simulink model "FSAE"  (R2023a)
settings: Solver=VariableStepAuto  StartTime=0.0  StopTime=1220  RelTol=1e-3
undefined symbols (not defined in the file): eta_EM_map, g, h, r_wheel, rho, T_EM_max, w_EM_row, w_EM_upper
settings Model: Creator=123ne  LastModifiedBy=123ne
settings ModelReferenceCC: EnableRefExpFcnMdlSchedulingChecks=on

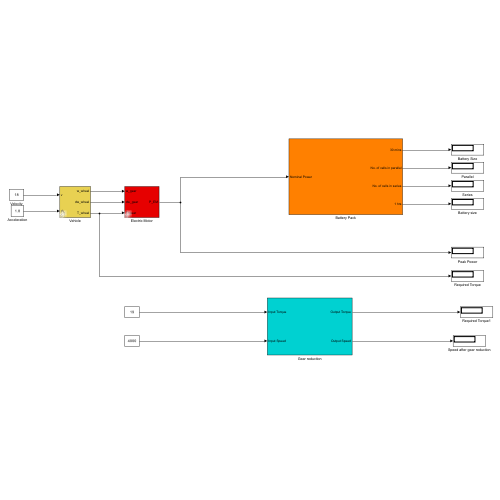
[thumbnail: Simulink's stored preview of the top-level diagram]
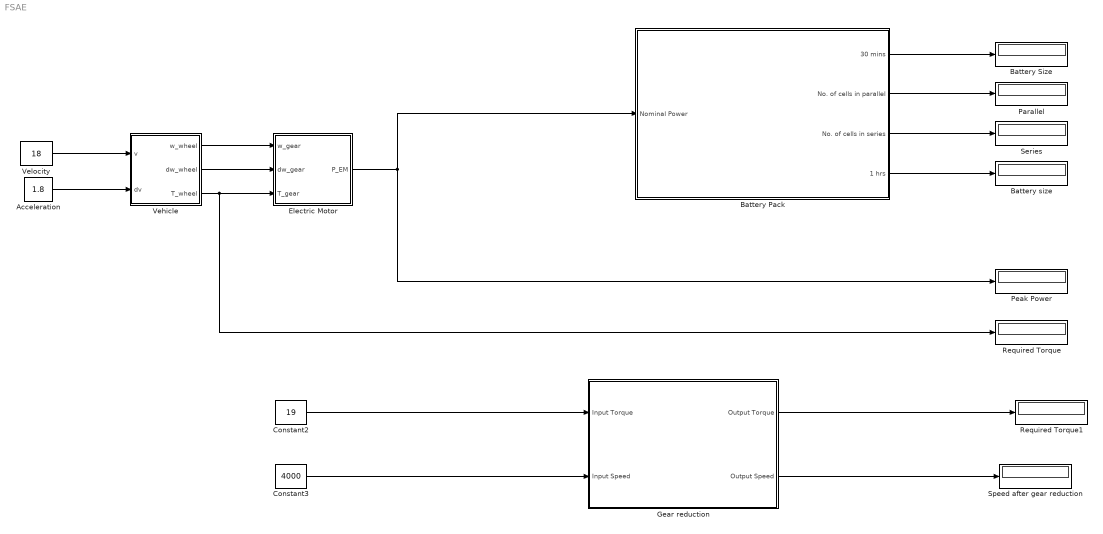
== system FSAE ==
  Acceleration : Constant  Value=1.8
  Battery Pack : Subsystem  mask{V_u=72, V_n=3.7}
      mask prompts: V_u "Specified Voltage"; V_n "Nominal Voltage"
  Battery Size : Display
  Battery size : Display
  Constant2 : Constant  Value=19
  Constant3 : Constant  Value=4000
  Electric Motor : Subsystem  AncestorBlock=qss_tb_library/Energy Converter/Electric Motor  mask(Electric Motor){scale_EM=1, theta_EM=0.1, P_aux=0}
      mask prompts: scale_EM "Motor scaling factor [-]"; theta_EM "Motor inertia [kg*m2]"; P_aux "Power required by auxiliaries [W]"
      mask help:
      | This block simulates the behaviour of an electric motor. The block is based on an efficiency map.
      |
      | Input:
      | =====
      | 	w_gear		Speed of the fly wheel [rad/s]
      | 	dw_gear	Acceleration of the fly wheel [rad/s^2]
      | 	T_gear		Torque on the fly wheel [Nm]
      |
      | Output:
      | ======
      | 	P_EM		Power produced by the electric motor [W]
      mask init:
      | init_EM;
      settings: LibrarySourceBlock=qss_tb_library/Energy Converter/Electric Motor
  Gear reduction : Subsystem  mask{r1=3.14, r2=4, r_1=3.14, r_2=4, R=0.507}
      mask prompts: r1 "Gear ratio"; r2 "Differential ratio"; r_1 "Gear ratio1"; r_2 "Differential ratio2"; R "radius"
  Parallel : Display
  Peak Power : Display
  Required Torque : Display
  Required Torque1 : Display
  Series : Display
  Speed after gear reduction : Display
  Vehicle : Subsystem  Tag=vehicle  AncestorBlock=qss_tb_library/Vehicle/Vehicle  mask(Vehicle){m_f=350, mt2m_f=5, A_f=0.35, d_wheel=0.507, cw=0.85, mu=0.018}
      mask prompts: m_f "Total mass of the vehicle [kg]"; mt2m_f "Rotating mass [%]"; A_f "Vehicle cross section [m^2]"; d_wheel "Wheel diameter [m]"; cw "Drag coefficient [-]"; mu "Rolling friction coefficient [-]"
      mask help:
      | This block computes the power required from the vehicle.
      |
      | Input:
      | =====
      | 	v		Speed [m/s]
      | 	dv		Acceleration [m/s^2]
      |
      | Output:
      | ======
      | 	w_wheel	Speed of the wheel [rad/s]
      | 	dw_wheel	Acceleration of the wheel [rad/s^2]
      | 	T_wheel	Torque on the wheel [Nm]
      mask init:
      | init_vehicle;
      settings: LibrarySourceBlock=qss_tb_library/Vehicle/Vehicle
  Velocity : Constant  Value=18
  wires:
  Vehicle/1(w_wheel) -> Electric Motor/1(w_gear)
  Vehicle/2(dw_wheel) -> Electric Motor/2(dw_gear)
  Vehicle/3(T_wheel) -> Electric Motor/3(T_gear), Required Torque/1
  Battery Pack/1(30 mins) -> Battery Size/1
  Battery Pack/2(No. of cells in parallel) -> Parallel/1
  Battery Pack/3(No. of cells in series) -> Series/1
  Battery Pack/4(1 hrs) -> Battery size/1
  Electric Motor/1(P_EM) -> Battery Pack/1(Nominal Power), Peak Power/1
  Constant2/1 -> Gear reduction/1(Input Torque)
  Gear reduction/1(Output Torque) -> Required Torque1/1
  Constant3/1 -> Gear reduction/2(Input Speed)
  Gear reduction/2(Output Speed) -> Speed after gear reduction/1
  Velocity/1 -> Vehicle/1(v)
  Acceleration/1 -> Vehicle/2(dv)

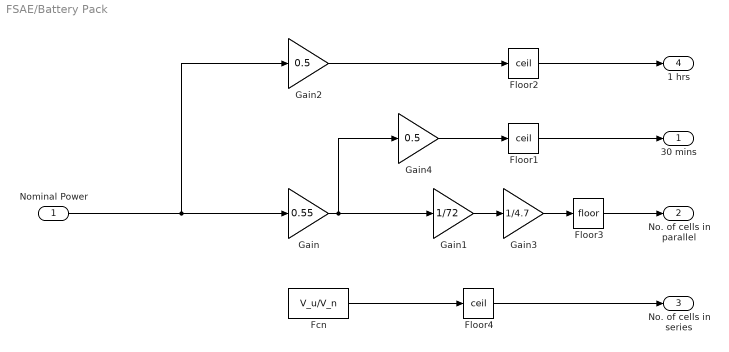
== system FSAE/Battery Pack ==
  Nominal Power : Inport
  Fcn : Fcn  Expr=V_u/V_n
  Floor1 : Rounding  Operator=ceil
  Floor2 : Rounding  Operator=ceil
  Floor3 : Rounding
  Floor4 : Rounding  Operator=ceil
  Gain : Gain  Gain=0.55
  Gain1 : Gain  Gain=1/72
  Gain2 : Gain  Gain=0.5
  Gain3 : Gain  Gain=1/4.7
  Gain4 : Gain  Gain=0.5
  30 mins : Outport
  No. of cells in parallel : Outport  Port=2
  No. of cells in series : Outport  Port=3
  1 hrs : Outport  Port=4
  wires:
  Gain/1 -> Gain1/1, Gain4/1
  Nominal Power/1 -> Gain2/1, Gain/1
  Gain1/1 -> Gain3/1
  Gain3/1 -> Floor3/1
  Floor1/1 -> 30 mins/1
  Fcn/1 -> Floor4/1
  Floor3/1 -> No. of cells in parallel/1
  Floor4/1 -> No. of cells in series/1
  Gain2/1 -> Floor2/1
  Floor2/1 -> 1 hrs/1
  Gain4/1 -> Floor1/1

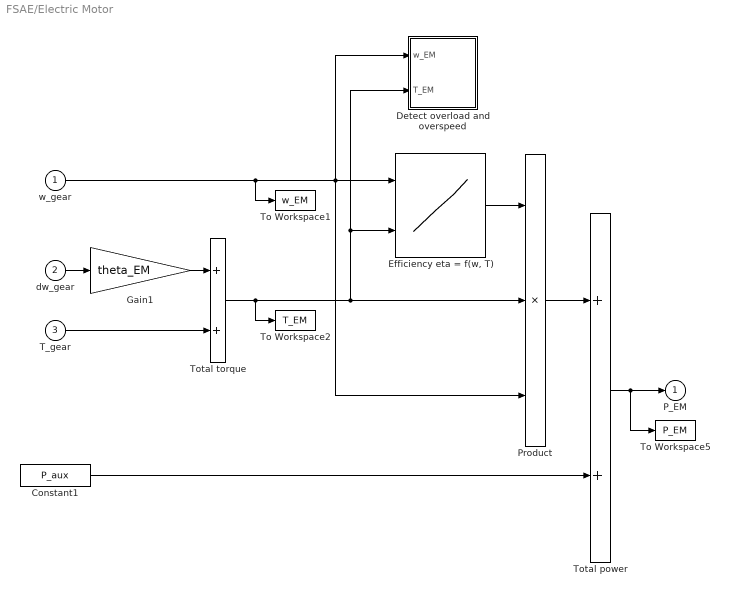
== system FSAE/Electric Motor ==
  w_gear : Inport
  dw_gear : Inport  Port=2
  T_gear : Inport  Port=3
  Constant1 : Constant  Value=P_aux
  Detect overload and overspeed : Subsystem
  "Efficiency eta = f(w, T)" : Lookup2D  RowIndex=w_EM_row  ColumnIndex=T_EM_col  Table=eta_EM_map  SaturateOnIntegerOverflow=off  InputSameDT=off
  Gain1 : Gain  Gain=theta_EM  SaturateOnIntegerOverflow=on  OutDataTypeStr=Inherit: Same as input  ParamDataTypeStr=Inherit: Same as input
  Product : Product  Inputs=3  InputSameDT=on  RndMeth=Zero  SaturateOnIntegerOverflow=on  OutDataTypeStr=Inherit: Same as first input
  To Workspace1 : ToWorkspace  VariableName=w_EM  SampleTime=-1
  To Workspace2 : ToWorkspace  VariableName=T_EM  SampleTime=-1
  To Workspace5 : ToWorkspace  VariableName=P_EM  SampleTime=-1
  Total power : Sum  InputSameDT=on  SaturateOnIntegerOverflow=on  OutDataTypeStr=Inherit: Same as first input
  Total torque : Sum  InputSameDT=on  SaturateOnIntegerOverflow=on  OutDataTypeStr=Inherit: Same as first input
  P_EM : Outport  InitialOutput=0
  wires:
  Total power/1 -> To Workspace5/1, P_EM/1
  Product/1 -> Total power/1
  Constant1/1 -> Total power/2
  Total torque/1 -> Product/2, "Efficiency eta = f(w, T)"/2, Detect overload and overspeed/2(T_EM), To Workspace2/1
  Gain1/1 -> Total torque/1
  T_gear/1 -> Total torque/2
  dw_gear/1 -> Gain1/1
  "Efficiency eta = f(w, T)"/1 -> Product/1
  w_gear/1 -> To Workspace1/1, Product/3, "Efficiency eta = f(w, T)"/1, Detect overload and overspeed/1(w_EM)

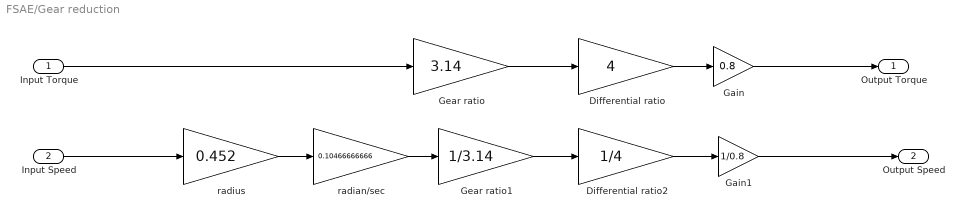
== system FSAE/Gear reduction ==
  Input Torque : Inport
  Input Speed : Inport  Port=2
  Differential ratio : Gain  Gain=4
  Differential ratio2 : Gain  Gain=1/4
  Gain : Gain  Gain=0.8
  Gain1 : Gain  Gain=1/0.8
  Gear ratio : Gain  Gain=3.14
  Gear ratio1 : Gain  Gain=1/3.14
  radian/sec : Gain  Gain=0.10466666666
  radius : Gain  Gain=0.452
  Output Torque : Outport
  Output Speed : Outport  Port=2
  wires:
  Gear ratio1/1 -> Differential ratio2/1
  Gear ratio/1 -> Differential ratio/1
  Input Torque/1 -> Gear ratio/1
  Input Speed/1 -> radius/1
  Differential ratio/1 -> Gain/1
  Differential ratio2/1 -> Gain1/1
  radius/1 -> radian/sec/1
  radian/sec/1 -> Gear ratio1/1
  Gain/1 -> Output Torque/1
  Gain1/1 -> Output Speed/1

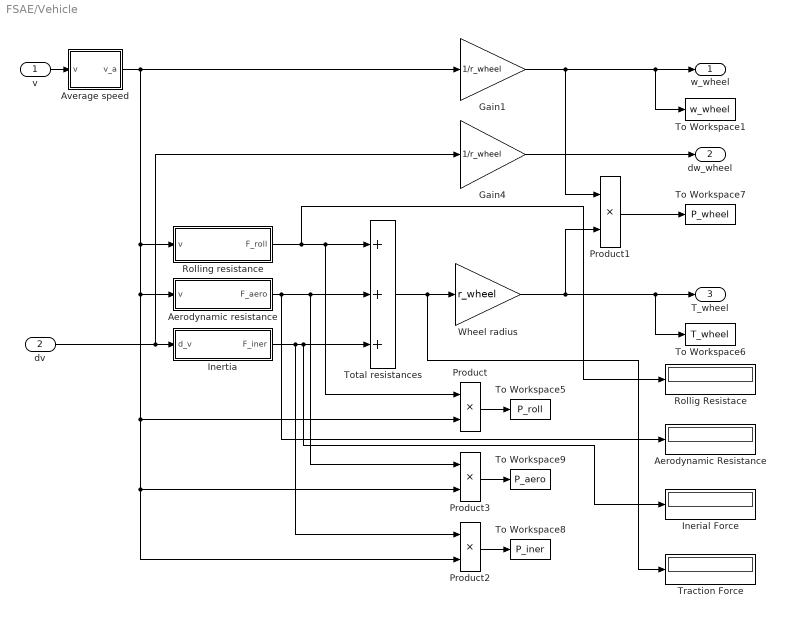
== system FSAE/Vehicle ==
  v : Inport
  dv : Inport  Port=2
  Aerodynamic Resistance : Display
  Aerodynamic resistance : Subsystem
  Average speed : Subsystem
  Gain1 : Gain  Gain=1/r_wheel  SaturateOnIntegerOverflow=on  OutDataTypeStr=Inherit: Same as input  ParamDataTypeStr=Inherit: Same as input
  Gain4 : Gain  Gain=1/r_wheel  SaturateOnIntegerOverflow=on  OutDataTypeStr=Inherit: Same as input  ParamDataTypeStr=Inherit: Same as input
  Inerial Force : Display
  Inertia : Subsystem
  Product{,1..3} (4 alike) : Product  InputSameDT=on  RndMeth=Zero  SaturateOnIntegerOverflow=on  OutDataTypeStr=Inherit: Same as first input
  Rollig Resistace : Display
  Rolling resistance : Subsystem
  To Workspace1 : ToWorkspace  VariableName=w_wheel  SampleTime=-1
  To Workspace5 : ToWorkspace  VariableName=P_roll  SampleTime=-1
  To Workspace6 : ToWorkspace  VariableName=T_wheel  SampleTime=-1
  To Workspace7 : ToWorkspace  VariableName=P_wheel  SampleTime=-1
  To Workspace8 : ToWorkspace  VariableName=P_iner  SampleTime=-1
  To Workspace9 : ToWorkspace  VariableName=P_aero  SampleTime=-1
  Total resistances : Sum  Inputs=+++  InputSameDT=on  SaturateOnIntegerOverflow=on  OutDataTypeStr=Inherit: Same as first input
  Traction Force : Display
  Wheel radius : Gain  Gain=r_wheel  SaturateOnIntegerOverflow=on  OutDataTypeStr=Inherit: Same as input  ParamDataTypeStr=Inherit: Same as input
  w_wheel : Outport  InitialOutput=0
  dw_wheel : Outport  Port=2  InitialOutput=0
  T_wheel : Outport  Port=3  InitialOutput=0
  wires:
  Product/1 -> To Workspace5/1
  Product1/1 -> To Workspace7/1
  Product3/1 -> To Workspace9/1
  Product2/1 -> To Workspace8/1
  v/1 -> Average speed/1(v)
  dv/1 -> Gain4/1, Inertia/1(d_v)
  Average speed/1(v_a) -> Rolling resistance/1(v), Product2/2, Product3/2, Product/2, Aerodynamic resistance/1(v), Gain1/1
  Wheel radius/1 -> To Workspace6/1, T_wheel/1, Product1/2
  Total resistances/1 -> Traction Force/1, Wheel radius/1
  Inertia/1(F_iner) -> Product2/1, Inerial Force/1, Total resistances/3
  Aerodynamic resistance/1(F_aero) -> Aerodynamic Resistance/1, Total resistances/2, Product3/1
  Rolling resistance/1(F_roll) -> Rollig Resistace/1, Product/1, Total resistances/1
  Gain1/1 -> To Workspace1/1, w_wheel/1, Product1/1
  Gain4/1 -> dw_wheel/1

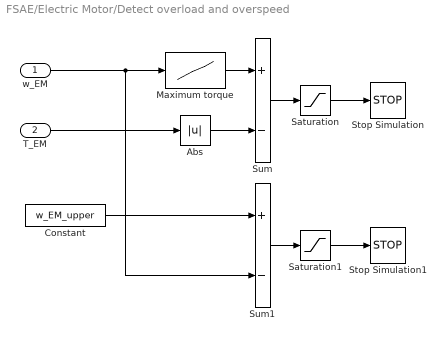
== system FSAE/Electric Motor/Detect overload and overspeed ==
  w_EM : Inport
  T_EM : Inport  Port=2
  Abs : Abs
  Constant : Constant  Value=w_EM_upper
  Maximum torque : Lookup  InputValues=w_EM_row  Table=T_EM_max
  Saturation : Saturate  UpperLimit=0  LowerLimit=-inf
  Saturation1 : Saturate  UpperLimit=0  LowerLimit=-inf
  Stop Simulation : Stop
  Stop Simulation1 : Stop
  Sum : Sum  Inputs=+-  InputSameDT=on  SaturateOnIntegerOverflow=on  OutDataTypeStr=Inherit: Same as first input
  Sum1 : Sum  Inputs=+-  InputSameDT=on  SaturateOnIntegerOverflow=on  OutDataTypeStr=Inherit: Same as first input
  wires:
  Sum/1 -> Saturation/1
  w_EM/1 -> Maximum torque/1, Sum1/2
  T_EM/1 -> Abs/1
  Maximum torque/1 -> Sum/1
  Abs/1 -> Sum/2
  Saturation/1 -> Stop Simulation/1
  Constant/1 -> Sum1/1
  Sum1/1 -> Saturation1/1
  Saturation1/1 -> Stop Simulation1/1

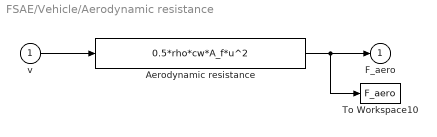
== system FSAE/Vehicle/Aerodynamic resistance ==
  v : Inport
  Aerodynamic resistance : Fcn  Expr=0.5*rho*cw*A_f*u^2
  To Workspace10 : ToWorkspace  VariableName=F_aero  SampleTime=-1
  F_aero : Outport  InitialOutput=0
  wires:
  Aerodynamic resistance/1 -> To Workspace10/1, F_aero/1
  v/1 -> Aerodynamic resistance/1

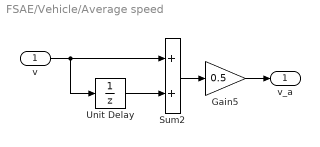
== system FSAE/Vehicle/Average speed ==
  v : Inport
  Gain5 : Gain  Gain=0.5  SaturateOnIntegerOverflow=on  OutDataTypeStr=Inherit: Same as input  ParamDataTypeStr=Inherit: Same as input
  Sum2 : Sum  InputSameDT=on  SaturateOnIntegerOverflow=on  OutDataTypeStr=Inherit: Same as first input
  Unit Delay : UnitDelay  SampleTime=h
  v_a : Outport  InitialOutput=0
  wires:
  v/1 -> Unit Delay/1, Sum2/1
  Gain5/1 -> v_a/1
  Sum2/1 -> Gain5/1
  Unit Delay/1 -> Sum2/2

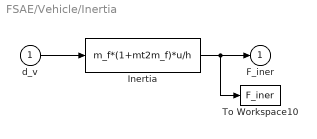
== system FSAE/Vehicle/Inertia ==
  d_v : Inport
  Inertia : Fcn  Expr=m_f*(1+mt2m_f)*u/h
  To Workspace10 : ToWorkspace  VariableName=F_iner  SampleTime=-1
  F_iner : Outport  InitialOutput=0
  wires:
  d_v/1 -> Inertia/1
  Inertia/1 -> To Workspace10/1, F_iner/1

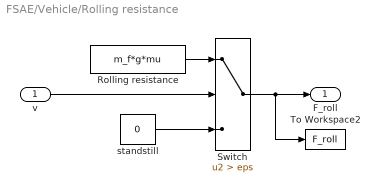
== system FSAE/Vehicle/Rolling resistance ==
  v : Inport
  Rolling resistance : Constant  Value=m_f*g*mu
  Switch : Switch  Criteria=u2 > Threshold  Threshold=eps  SaturateOnIntegerOverflow=off  InputSameDT=off
  To Workspace2 : ToWorkspace  VariableName=F_roll  SampleTime=-1
  standstill : Constant  Value=0
  F_roll : Outport
  wires:
  Rolling resistance/1 -> Switch/1
  standstill/1 -> Switch/3
  v/1 -> Switch/2
  Switch/1 -> F_roll/1, To Workspace2/1
